simulink model "part2_3"  (R2018b)
settings: Solver=VariableStepAuto  StartTime=0.0  StopTime=100  MaxStep=0.01*0.1551  RelTol=1e-3
settings Model: Creator=buddyugwumba1  LastModifiedBy=buddyugwumba1

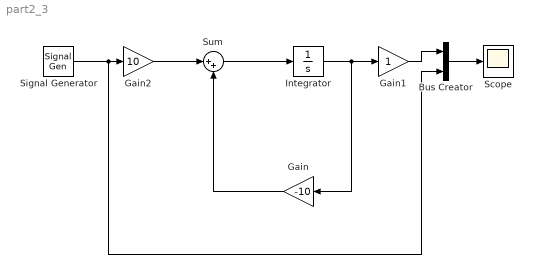
== system part2_3 ==
  Bus Creator : BusCreator  Inputs=2
  Gain : Gain  Gain=-10
  Gain1 : Gain
  Gain2 : Gain  Gain=10
  Integrator : Integrator
  Scope : Scope
  Signal Generator : SignalGenerator  Units=rad/sec
  Sum : Sum  Inputs=|++
  wires:
  Bus Creator/1 -> Scope/1
  Signal Generator/1 -> Bus Creator/2, Gain2/1
  Gain2/1 -> Sum/1
  Sum/1 -> Integrator/1
  Integrator/1 -> Gain/1, Gain1/1
  Gain1/1 -> Bus Creator/1
  Gain/1 -> Sum/2
